simulink model "AmplitudeModulation"  (R2023b)
settings: Solver=VariableStepAuto  StartTime=0.0  StopTime=5.0  RelTol=1e-3
settings Model: Creator=satyamagrawal  LastModifiedBy=dariksha

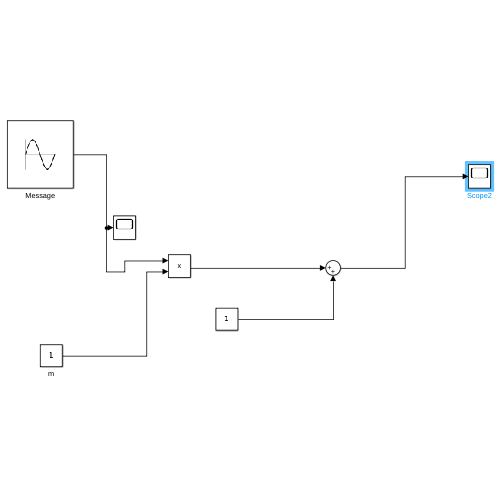
[thumbnail: Simulink's stored preview of the top-level diagram]
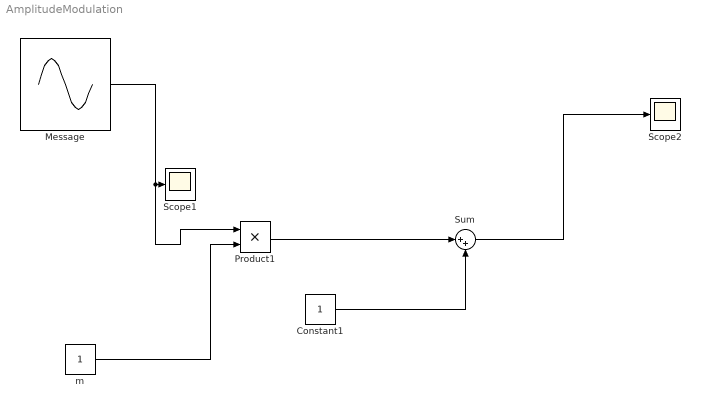
== system AmplitudeModulation ==
  Constant1 : Constant
  Message : Sin  Amplitude=3  Frequency=314.159265  SampleTime=0
  Product1 : Product
  Scope1 : Scope
  Scope2 : Scope
  Sum : Sum  Inputs=|++
  m : Constant
  wires:
  Message/1 -> Product1/1, Scope1/1
  m/1 -> Product1/2
  Product1/1 -> Sum/1
  Constant1/1 -> Sum/2
  Sum/1 -> Scope2/1
